simulink model "SRManCw1_PM2R_MODEL"  (R2018a)
settings: Solver=VariableStepAuto  StartTime=0.0  StopTime=10.0  RelTol=1e-3
values from neighbouring files (symbols this model uses):
  Qd1 = 0.2    [ZAD1_Init.m]
  Qd2 = 0.3    [ZAD1_Init.m]
undefined symbols (not defined in the file or in its folder): w
settings Model: Creator=szymon  LastModifiedBy=szymon

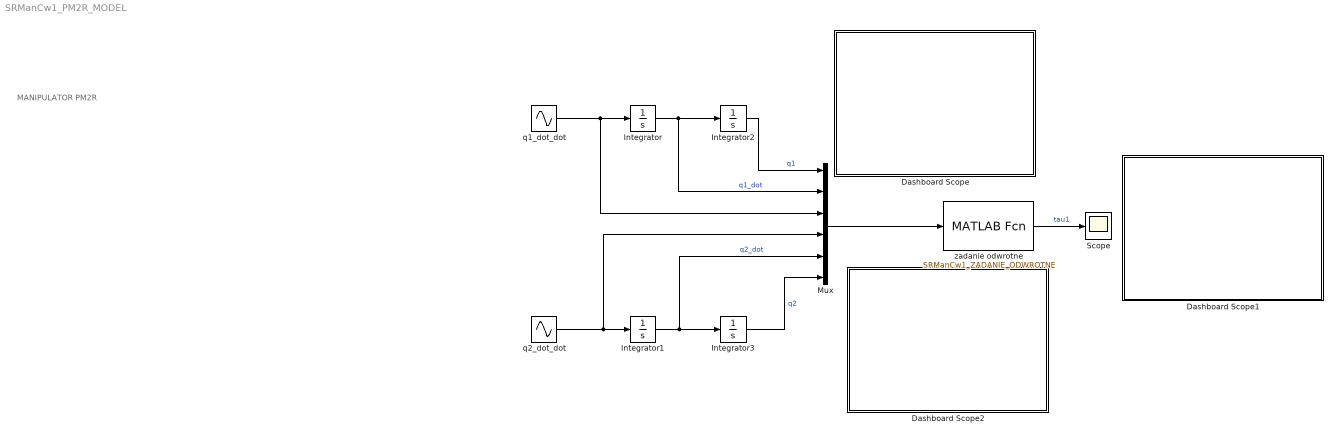
== system SRManCw1_PM2R_MODEL ==
  note: MANIPULATOR PM2R
  Dashboard Scope : Subsystem  DialogController=hmiCreateDDGDialog  IsWebBlock=on  mask(MWDashboardBlock){webBlockId=85f042bb-43e3-417a-a2e5-29409c83120d, webBlockType=sdiscope, ShowInitialText=on, HMISrcModelName=SRManCw1_PM2R_MODEL}
      mask prompts: webBlockId "WebBlock Id"; webBlockType "WebBlock Type"; HMISrcModelName "Source Model"
      mask help: SimulinkHMI:dialogs:HMIScopeDialogDesc
      mask Help: helpview([docroot '/mapfiles/simulink.map'], 'hmi_scope')
      mask Display:
      | if strcmp(get_param(bdroot(gcb),'BlockDiagramType'), 'library')
      |     image([(matlabroot) '/toolbox/simulink/hmi/icons/DashboardScope.png']);
      | end
  Dashboard Scope1 : Subsystem  DialogController=hmiCreateDDGDialog  IsWebBlock=on  mask(MWDashboardBlock){webBlockId=cd777eac-a354-456c-9f5d-ab5ff5201cfb, webBlockType=sdiscope, ShowInitialText=on, HMISrcModelName=SRManCw1_PM2R_MODEL}
      mask prompts: webBlockId "WebBlock Id"; webBlockType "WebBlock Type"; HMISrcModelName "Source Model"
      mask help: SimulinkHMI:dialogs:HMIScopeDialogDesc
      mask Help: helpview([docroot '/mapfiles/simulink.map'], 'hmi_scope')
      mask Display:
      | if strcmp(get_param(bdroot(gcb),'BlockDiagramType'), 'library')
      |     image([(matlabroot) '/toolbox/simulink/hmi/icons/DashboardScope.png']);
      | end
  Dashboard Scope2 : Subsystem  DialogController=hmiCreateDDGDialog  IsWebBlock=on  mask(MWDashboardBlock){webBlockId=b849867b-a4a0-4224-a1ea-8274c603c54b, webBlockType=sdiscope, ShowInitialText=on, HMISrcModelName=SRManCw1_PM2R_MODEL}
      mask prompts: webBlockId "WebBlock Id"; webBlockType "WebBlock Type"; HMISrcModelName "Source Model"
      mask help: SimulinkHMI:dialogs:HMIScopeDialogDesc
      mask Help: helpview([docroot '/mapfiles/simulink.map'], 'hmi_scope')
      mask Display:
      | if strcmp(get_param(bdroot(gcb),'BlockDiagramType'), 'library')
      |     image([(matlabroot) '/toolbox/simulink/hmi/icons/DashboardScope.png']);
      | end
  Integrator{,1..3} (4 alike) : Integrator
  Mux : Mux  Inputs=6
  Scope : Scope
  "q1_dot_dot " : Sin  Amplitude=-w^2*Qd1  SampleTime=0
  "q2_dot_dot " : Sin  Amplitude=-w^2*Qd2  SampleTime=0
  zadanie odwrotne : MATLABFcn  MATLABFcn=SRManCw1_ZADANIE_ODWROTNE
  wires:
  "q2_dot_dot "/1 -> Mux/4, Integrator1/1
  Integrator1/1 -> Mux/5, Integrator3/1  "q2_dot"
  "q1_dot_dot "/1 -> Mux/3, Integrator/1
  Integrator/1 -> Mux/2, Integrator2/1  "q1_dot"
  Integrator2/1 -> Mux/1  "q1"
  Integrator3/1 -> Mux/6  "q2"
  zadanie odwrotne/1 -> Scope/1  "tau1"
  Mux/1 -> zadanie odwrotne/1

== system SRManCw1_PM2R_MODEL/Dashboard Scope ==

== system SRManCw1_PM2R_MODEL/Dashboard Scope1 ==

== system SRManCw1_PM2R_MODEL/Dashboard Scope2 ==
